simulink model "LQR"  (R2015a)
settings: Solver=ode45  StartTime=0.0  StopTime=10.0  RelTol=1e-3
values from neighbouring files (symbols this model uses):
  A = [3.3545 -4.3521 2.6058 -0.6082; 1 0 0 0; 0 1 0 0; 0 0 1 0]    [LQGm.m]    (also in Testes_planta.m = [3.11506910744011 -3.74010634305672 2.06382118501694 -0.4387)
  B = [1;0;0;0]    [LQGm.m]    (also in Testes_planta.m)
  C = [-0.0657 0.1152 0 0]    [LQGm.m]    (also in Testes_planta.m = [-0.0767099115028891 0.161398714293952 0 0])
undefined symbols (not defined in the file or in its folder): K
settings Model: Creator=user  LastModifiedBy=user

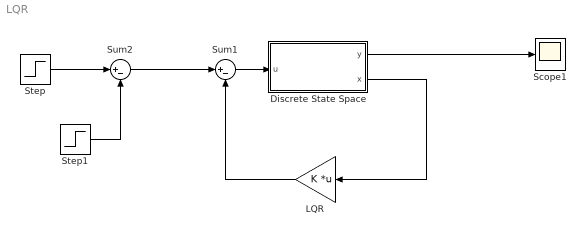
== system LQR ==
  "Discrete State Space " : Subsystem
  LQR : Gain  Gain=K  Multiplication=Matrix(K*u)
  Scope1 : Scope
  Step : Step  Time=0  SampleTime=0
  Step1 : Step  SampleTime=0
  Sum1 : Sum  Inputs=|+-
  Sum2 : Sum  Inputs=|+-
  wires:
  "Discrete State Space "/1(y) -> Scope1/1
  "Discrete State Space "/2(x) -> LQR/1
  LQR/1 -> Sum1/2
  Sum1/1 -> "Discrete State Space "/1(u)
  Sum2/1 -> Sum1/1
  Step/1 -> Sum2/1
  Step1/1 -> Sum2/2

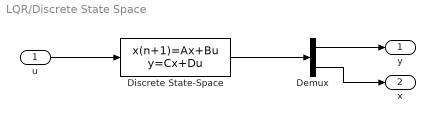
== system LQR/Discrete State Space  ==
  u : Inport
  Demux : Demux  Outputs=[1 length(A)]
  Discrete State-Space : DiscreteStateSpace  A=A  B=B  C=[C;eye(4)]  D=[0;0;0;0;0]  SampleTime=0.02
  y : Outport
  x : Outport  Port=2
  wires:
  Discrete State-Space/1 -> Demux/1
  Demux/1 -> y/1
  Demux/2 -> x/1
  u/1 -> Discrete State-Space/1
